simulink model "Model_TranslationEngine64"  (R2022b)
settings: Solver=FixedStepDiscrete  StartTime=0.0  StopTime=5  RelTol=1e-3  EnableMultiTasking=on
InitFcn:
  | % Initialize model
  | ModelSettings=BTConfig.GetModelSettings();
  | 
  | ModelSettings.Validate();
  | 
  | ModelInit;
  | 
  | 
  | % load library data
  | GainLibrary_data;
  | % Load saved values from partition process
  | CapturedConstMask.LoadMapFromFile(bdroot)
StartFcn:
  | % make sure all the simulated RTC requests are found
  | %RTC_SIM_OBJ.ValidateREQs();
undefined symbols (not defined in the file or in its folder): AA, BPLP, Column, NumHFRefBPF, NumHFRefLPF, NumMusicChannels, Row, VolumeMuteConfig
libraries: TuneVar x925, TOP x490, FeaturePath x111, CapturedConstLib x52
(part 1 of 34)
settings Model: Creator=kl13806  LastModifiedBy=mp55777
settings DataIOCC: ReturnWorkspaceOutputs=off
settings OptimizationCC: DefaultParameterBehavior=Inlined  DefaultUnderspecifiedDataType=single  EfficientTunableParamExpr=on
settings DebuggingCC: MergeDetectMultiDrivingBlocksExec=none  InheritedTsInSrcMsg=none  MultiTaskDSMMsg=none  ParameterPrecisionLossMsg=none  ParameterTunabilityLossMsg=error  UnconnectedInputMsg=warning  UnconnectedOutputMsg=warning  UnconnectedLineMsg=warning  UnknownTsInhSupMsg=none  SFUnexpectedBacktrackingDiag=warning  SFNoUnconditionalDefaultTransitionDiag=warning  SFExecutionAtInitializationDiag=none  SFMachineParentedDataDiag=warning
settings HardwareCC: ProdBitPerPointer=32  ProdBitPerSizeT=32  ProdBitPerPtrDiffT=32  ProdWordSize=32  ProdHWDeviceType=Intel->x86-32 (Windows32)  TargetBitPerPointer=64  TargetBitPerSizeT=64  TargetBitPerPtrDiffT=64  TargetLongLongMode=on  TargetIntDivRoundTo=Zero  TargetEndianess=LittleEndian  TargetWordSize=64  TargetHWDeviceType=MATLAB Host  ProdEqTarget=off
settings ModelReferenceCC: EnableRefExpFcnMdlSchedulingChecks=on  ModelReferenceNumInstancesAllowed=Single
settings SFSimCC: MATLABDynamicMemAlloc=off
settings RTWCC: Description=Embedded Coder (host-based shared library target)  SystemTargetFile=ert_shrlib.tlc  TLCOptions="-aTALARIA_ENGINE=\"Translation\""  TemplateMakefile=ert_default_tmf  RTWVerbose=off  RetainRTWFile=on  Toolchain=MinGW64 | gmake (64-bit Windows)  IncludeHyperlinkInReport=on
settings RTWCC: CustomHeaderCode=|
  | // Auto-generated code for model Model
  | /**** TOP TOKEN COMPATIBILITY HASH VALUES ****/
  | #define TOP_COMPAT {0x21D75357UL, 0x72F610E9UL, 0x8E520967UL, 0x8735CAA1UL, 0x168A3EA6UL}
  | #define TOP_COMPAT_NAME {"InputSelect", "PreAmp", "Near", "PostProcess", "TestRouter"}
  | #define TOP_COMPAT_NAME_HASH {0xF8044409UL, 0xC3A89EEBUL, 0xD67EB32FUL, 0x062DAD3BUL, 0x8CC5BE54UL}
  | /**** COMPAT HASH VALUES BY MODULE ****/
  | #define INPUTSELECT_TOP_COMPAT 0x21D75357UL
  | #define PREAMP_TOP_COMPAT 0x72F610E9UL
  | #define NEAR_TOP_COMPAT 0x8E520967UL
  | #define POSTPROCESS_TOP_COMPAT 0x8735CAA1UL
  | #define TESTROUTER_TOP_COMPAT 0x168A3EA6UL
  | /**** NAME HASH VALUES BY MODULE ****/
  | #define INPUTSELECT_TOP_NAME_HASH 0xF8044409UL
  | #define PREAMP_TOP_NAME_HASH 0xC3A89EEBUL
  | #define NEAR_TOP_NAME_HASH 0xD67EB32FUL
  | #define POSTPROCESS_TOP_NAME_HASH 0x062DAD3BUL
  | #define TESTROUTER_TOP_NAME_HASH 0x8CC5BE54UL
settings CodeAppCC: ForceParamTrailComments=on  IgnoreCustomStorageClasses=off  MaxIdLength=128  OperatorAnnotations=on  SimulinkDataObjDesc=on  SFDataObjDesc=on  MATLABFcnDesc=on  InsertBlockDesc=on  StateflowObjectComments=on  MATLABSourceComments=on
settings STFCustomTargetCC: TargetLangStandard=C99 (ISO)  MultiwordLength=256  ParMdlRefBuildCompliant=on  CompOptLevelCompliant=on  CombineOutputUpdateFcns=on  ERTCustomFileBanners=on  SupportContinuousTime=off  SupportNonInlinedSFcns=off  RemoveResetFunc=on  SupportVariableSizeSignals=on  MATLABClassNameForMDSCustomization=Simulink.SoftwareTarget.ERTCustomization  ModelStepFunctionPrototypeControlCompliant=on  UseToolchainInfoCompliant=on  SystemTargetFile=ert_shrlib.tlc
settings ERTTargetCC: TargetLangStandard=C99 (ISO)  ConcurrentExecutionCompliant=off  SupportVariableSizeSignals=on  CPPClassGenCompliant=off  InlinedParameterPlacement=NonHierarchical  ERTCustomFileTemplate=translation_dll.tlc  IndentStyle=Allman  IndentSize=4

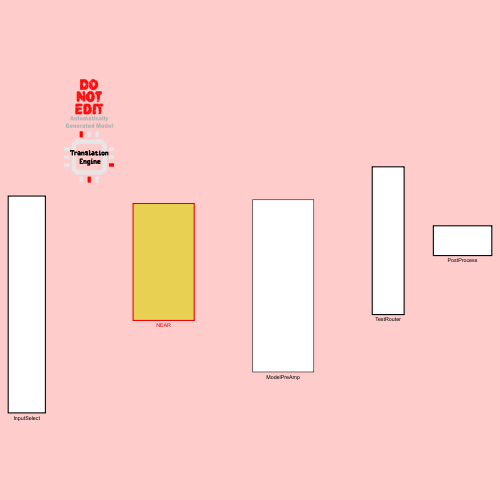
[thumbnail: Simulink's stored preview of the top-level diagram]
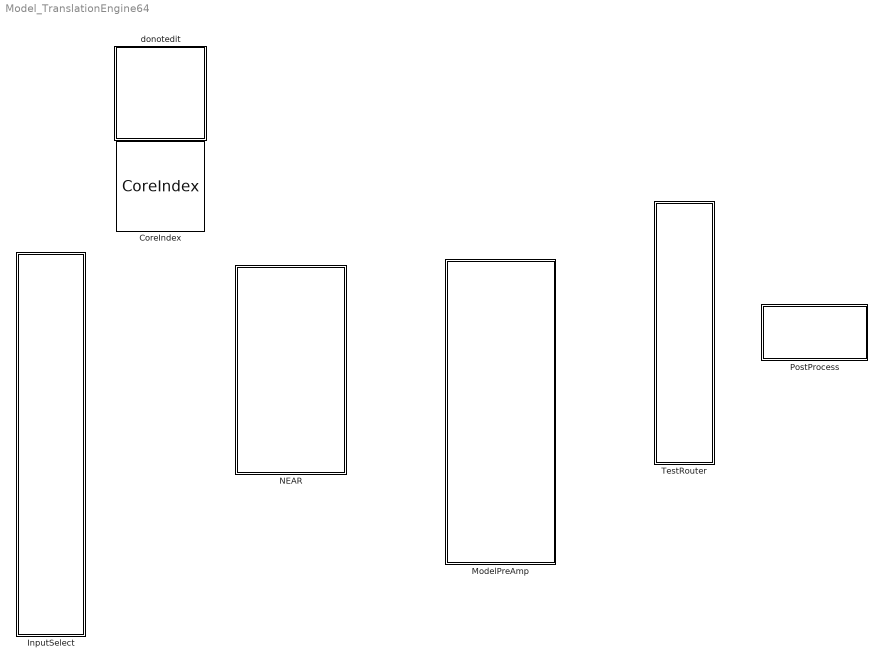
== system Model_TranslationEngine64 ==
  CoreIndex : FeaturePath/CoreIndex  Role=Translation Engine  CoreIndex=9  Config=[]  AddressingMode=Indirect core determination via table lookup (i.e. use Partition blocks)  CrossCoreApi=None  CrossCoreAllocation=None  CrossCoreSampleTime=-1  BasePeriod=[]  TriggerInit=[440 234 535 331]
      settings: SourceProductName=Bose Talaria
  InputSelect : Subsystem  TreatAsAtomicUnit=on  mask{Config=ModelSettings.InputSelect}
      mask prompts: Config "InputSelectConfig"
      settings: RTWSystemCode=Nonreusable function
  ModelPreAmp : Subsystem  mask{Config=ModelSettings.ModelPreAmp}
      mask prompts: Config "PreAmpConfig"
  NEAR : Subsystem  TreatAsAtomicUnit=on  mask{Config=ModelSettings.NearConfig}
      mask prompts: Config "NearConfig"
  PostProcess : Subsystem  TreatAsAtomicUnit=on  mask{Config=ModelSettings.PostProcess}
      mask prompts: Config "PostProcessConfig"
  TestRouter : Subsystem  TreatAsAtomicUnit=on  mask{Config=ModelSettings.TestRouter}
      mask prompts: Config "TestRouterConfig"
  donotedit : Subsystem
      settings: OpenFcn=Model
      mask Display: image('DoNotEdit.svg');

== system Model_TranslationEngine64/InputSelect ==
  FeaturePath : FeaturePath/FeaturePath  FeatureName=InputSelect  IsGroup=on  GroupNumber=0  IsModule=on  TriggerInit=[105 216 220 329]
      settings: SourceProductName=Bose Talaria
  Router : Subsystem  mask(Blocklib Router){Config=Config.RouterCfg, FeatureName=RouterCfg}
      mask prompts: Config "RouterConfig"; FeatureName "Feature path name:"
      mask help: This block allows the user to route X input channels to Y output channels. Enter a value of 0 to "zero out" the specific channel
      mask init:
      | blkh=gcbh;
      | Config=BTConfig.Assert(blkh,Config);
      | 
      | Config.Validate();
      | BTConfig.InitSetFeatureIfPresent(blkh,'FeatureName');
      mask Callback Config: BTConfig.CallbackHideIfPresent(gcbh,{'FeatureName'});
      mask TypeOptions FeatureName: FeaturePath/FeatureName
      mask Display: image('routerIcon.png');

== system Model_TranslationEngine64/ModelPreAmp ==
  DecRate : Subsystem
  FeaturePath : FeaturePath/FeaturePath  FeatureName=PreAmp  IsGroup=on  GroupNumber=2  IsModule=on  TriggerInit=[-135 -246 -20 -139]
      settings: SourceProductName=Bose Talaria
  PreAmpPart1 : Subsystem  TreatAsAtomicUnit=on
      settings: RTWSystemCode=Nonreusable function  FunctionWithSeparateData=on

== system Model_TranslationEngine64/NEAR ==
  FeaturePath : FeaturePath/FeaturePath  FeatureName=Near  IsGroup=on  GroupNumber=1  IsModule=on  TriggerInit=[15 -306 130 -199]
      settings: SourceProductName=Bose Talaria
  Near1p1 : Subsystem  mask{Config=Config.Near}
      mask prompts: Config "Near1p1Config"
      mask init:
      | blkh=gcbh;
      | Config=BTConfig.Assert(blkh,Config);
      | % sample_rate_in_hertz                        = near.sample_rate_in_hertz;
      | % frame_size                                  = near.frame_size;
      | % ann_sysin_channel_count                     = near.ann_sysin_channel_count;
      | % front_peripheral_channel_count              = near.front_peripheral_channel_count;
      | % NEAR1p1FrontPeripheralChannelCountFullRate  = near.NEAR1p1FrontPeripheralChannelCountFullRate;
      | % NearWbAnnCount                              = near.NearWbAnnCount;
      | % headrest_count                              = near.headrest_count;
      | % channels_per_headrest                       = near.channels_per_headrest;
      | % decimation_factor                           = near.decimation_factor;
      | % rear_channel_count                          = near.rear_channel_count;
      | % vm                                          = near.vm;
      | % decimated_frame_size                        = near.decimated_frame_size;
      | % decimated_sample_rate_in_hertz              = near.decimated_sample_rate_in_hertz;
      | Config.Validate();
      | Config.DoMaskInit(blkh);

== system Model_TranslationEngine64/PostProcess ==
  FeaturePath : FeaturePath/FeaturePath  FeatureName=PostProcess  IsGroup=on  GroupNumber=3  IsModule=on  TriggerInit=[85 -186 200 -79]
      settings: SourceProductName=Bose Talaria
  PostProcess : Subsystem  TreatAsAtomicUnit=on
      settings: RTWSystemCode=Nonreusable function  RTWFcnNameOpts=Use subsystem name  RTWFileNameOpts=Use subsystem name  FunctionWithSeparateData=on

== system Model_TranslationEngine64/TestRouter ==
  ASDRouter : Subsystem  mask{frameSize=Config.FrameSize, nChanOut=Config.NumChanOut, mainSelect=Config.MainSelect, numMainCh=Config.NumMainCh, mainGain=Config.MainGain, enableAux=Config.EnableAux, numAux=Config.NumAux, auxGain=Config.AuxGain}
      mask prompts: frameSize "Frame Size (L)"; nChanOut "Number of Output Channels"; mainSelect "Main Channel Select Vector"; numMainCh "Number of Main Channels"; mainGain "Main gain for each output channel"; enableAux "Enable Aux input sources"; numAux "Number of Aux Channels"; auxGain "Aux gain for each output channel for each Aux source"
      mask init:
      | blkh = gcbh;
      | % Copy discrete mask parameters into a classdef object
      | InnerLinkConfig = AsdRouterConfig;
      | InnerLinkConfig.FrameSize = frameSize;
      | InnerLinkConfig.NumChanOut = nChanOut;
      | InnerLinkConfig.MainSelect = mainSelect;
      | InnerLinkConfig.NumMainCh = numMainCh;
      | InnerLinkConfig.MainGain = mainGain;
      | InnerLinkConfig.EnableAux = enableAux;
      | InnerLinkConfig.NumAux = numAux;
      | InnerLinkConfig.AuxGain = auxGain;
  FeaturePath : FeaturePath/FeaturePath  FeatureName=TestRouter  IsGroup=on  GroupNumber=5  IsModule=off  TriggerInit=[290 -166 405 -59]
      settings: SourceProductName=Bose Talaria
  TuneTOP : Subsystem  mask(Talaria Trivial Tune TOP){TriggerInit=[175 117 345 173], TopName=AuxSelect, TuneName=AuxSelect, DataTypeOut=int32, MaskValue=Config.MainGain, TunabilityNumber=1, MinValue=[], MaxValue=[], BankNumber=0, PreOverlay=false, PostOverlay=false, UseSameName=on}
      mask prompts: TriggerInit "Hidden: MoveFcn redraw"; TopName "Name:"; TuneName "Name of TuneVar:"; DataTypeOut "Data type:"; MaskValue "Default Value:"; TunabilityNumber "Tunability:"; MinValue "Min Value:"; MaxValue "Max Value:"; BankNumber "Target memory bank number:"; PreOverlay "Requires pre-overlay action:"; PostOverlay "Requires post-overlay action:"; UseSameName "Use same name for tune variable and TOP"
      mask help: The TuneTOP block encapsultes a Target Overlay Parameter, a Tune Variable, and a Trivial Translation between them.
      mask init:
      | [ok,activeTopPath,activeTunePath] = TuneTOP_Mask.Init(gcbh);
      settings: MoveFcn=TuneTOP_Mask.CB_TriggerInit(gcbh);
      mask Callback TriggerInit: TuneTOP_Mask.CB_TriggerInit(gcbh);
      mask TypeOptions TopName: TOP/TopName
      mask TypeOptions TuneName: Tune Variable/TuneName
      mask TypeOptions DataTypeOut: TOP/DataTypeOut
      mask TypeOptions MaskValue: Tune Variable/MaskValue
      mask TypeOptions TunabilityNumber: Tune Variable/TunabilityNumber
      mask Callback TunabilityNumber: TuneVarMask.CB_TunabilityNumber(gcbh);
      mask TypeOptions MinValue: Tune Variable/MinValue
      mask TypeOptions MaxValue: Tune Variable/MaxValue
      mask TypeOptions BankNumber: TOP/BankNumber
      mask TypeOptions PreOverlay: TOP/PreOverlay
      mask TypeOptions PostOverlay: TOP/PostOverlay
      mask Callback UseSameName: TuneTOP_Mask.CB_UseSameName(gcbh);
      mask DialogControl toolPanel Prompt: Tuning Tool Hints
      mask DialogControl DescriptionGroup Prompt: Description
      mask DialogControl EditDescription Prompt: Edit Description
      mask DialogControl EditDescription Callback: TuneTOP_Mask.CB_EditDescription(gcbh);
      mask DialogControl TunabilityText Prompt: Easy: Changes nearly every tuning.
      mask DialogControl AdvancedPanel Prompt: Advanced
      mask DialogControl ConvertToFullTranslation Prompt: Irreversible conversion to full translation
      mask DialogControl ConvertToFullTranslation Callback: TuneTOP_Mask.CB_ConvertToFullTranslation(gcbh);
      mask DialogControl ErrorContainer Prompt: Error Messages
      mask DialogControl ErrorText Prompt: Default value cannot be empty. Tune variables must have non-zero dimensions.
      mask Display:
      | % retrieve icon definition
      | [path,w,h] = TuneTOP_Mask.Icon();
      | 
      | % retrieve the block's pixel size
      | pos = get(gcbh,'position');
      | bw = pos(3) - pos(1);
      | bh = pos(4) - pos(2);
      | 
      | % draw centered icon
      | xAdj = bw/2 - w/2 + 5;
      | yAdj = bh/2 - h/2 + 4;
      | for i=1:length(path)
      | 	patch(path(i).x+xAdj, path(i).y+yAdj, path(i).rgb);
      | end
      | 
      | % show the top name or an X
      | if (exist('ok','var') && ok)
      | 	text(bw*0.5, bh*0.2, activeTopPath, 'horizontalAlignment', 'center');
      | 	patch(0,0,[1 1 1]);
      | 	patch(bw,bh,[1 1 1]);
      | else
      | 	tx=bw*0.03;
      | 	ty=bh*0.03;
      | 	patch([0 tx bw bw-tx], [ty 0 bh-ty bh], [1 0 0]);
      | 	patch([0 bw-tx bw tx], [bh-ty 0 ty bh], [1 0 0]);
      | end

== system Model_TranslationEngine64/donotedit ==

== system Model_TranslationEngine64/InputSelect/Router ==
  FeaturePath : FeaturePath/FeaturePath  FeatureName=RouterCfg  IsGroup=off  GroupNumber=-1  IsModule=off  TriggerInit=[615 164 730 271]
      settings: SourceProductName=Bose Talaria
  TOP : TOP/TOP  TriggerInit=[660 425 805 485]  TopName=OutMap  DataTypeOut=int32  BankNumber=0  PreOverlay=false  PostOverlay=false  Role=Automatic
      settings: SourceProductName=Bose Talaria
  TranslateTrigger : TuneVar/TranslateTrigger  TriggerInit=[526 305 564 360]
      settings: SourceProductName=Bose Talaria
  Trivial Translation : MATLAB Function  TreatAsAtomicUnit=on  mask{nInRouterMask=Config.NumIn}
      mask prompts: nInRouterMask "Num Input"
  TuneVarRouterMap : TuneVar/TuneVar  TuneName=Map  SpecifyMaxSize=on  VariableDim=2 (Column)  MaxSize=[1 Config.NumOut]  TunabilityNumber=1  MinValue=[]  MaxValue=[]  TriggerInit=[250 430 420 480]  MaskValue=Config.DefaultOutputMap
      settings: SourceProductName=Bose Talaria
  wires:
  TranslateTrigger/1 -> Trivial Translation/Trigger
  Trivial Translation/1(OutMap) -> TOP/1
  TuneVarRouterMap/1 -> Trivial Translation/1(Map)  "Map"

== system Model_TranslationEngine64/ModelPreAmp/DecRate ==
  AudioPilot35 : Subsystem  TreatAsAtomicUnit=on
      settings: RTWFcnNameOpts=Use subsystem name  RTWFileNameOpts=Use subsystem name  FunctionWithSeparateData=on
  Medusa5H1 : Subsystem

== system Model_TranslationEngine64/ModelPreAmp/PreAmpPart1 ==
  Bass : Subsystem  mask(Blocklib Tone){FeatureName=Bass, Config=Config.Bass, TriggerInit=[215 80 320 140]}
      mask prompts: FeatureName "Feature path name:"; Config "ToneConfig"; TriggerInit "Hidden: MoveFcn redraw"
      mask help: The tone block performs the treble and bass tone controls across multiple channels via a 1st order filter.
      mask init:
      | blkh=gcbh;
      | Config=BTConfig.Assert(blkh,Config);
      | 
      | BTConfig.InitSetFeatureIfPresent(blkh,'FeatureName');
      | Config.Validate();
      | ToneMask.Init(blkh);
      mask Help:
      | The tone block performs the treble and bass tone controls across multiple channels via a 1st order filter. The treble/ bass content can either be 'boosted' or 'cut' depending on the value of the gain. Different filters can be used for the boost and cut regions, each with its own cut-off frequency.
      | 
      | MASK PARAMETERS:
      | - Different filter coefficients can be applied for the boost and cut regions
      | - The maximum boost/ cut can be specified (typically 20 dB and -20 dB)
      | - The offset and scale values determine the piecewise linear curve that maps the index to the gain (typically 128 and 127 respectively)
      | 
      | RTC CONTROL:
      | Run time control is available to dynamically change the gain to be applied to the treble/bass content. An index (typically between 0-255) can be provided along with a ramp time and rate (rate gets precedence).
      | RTC_SIM_OBJ.AddREQ( 'TrebleBassSet', 0.6, [0005,  <tone_index>, <ramp_db_per_second>, <ramp_time>]);
      | E.g., RTC_SIM_OBJ.AddREQ( 'TrebleBassSet', 0.6, [0005,  50, 0, 50]);
      mask TypeOptions FeatureName: FeaturePath/FeatureName
      mask Callback Config: BTConfig.CallbackHideIfPresent(gcbh,{'FeatureName'});
      mask Callback TriggerInit: ToneMask.CB_TriggerInit(gcbh);
      mask Display:
      | [path w h] = IconToneMask();
      | 
      | % retrieve the block's pixel size
      | pos = get(gcbh,'position');
      | bw = pos(3) - pos(1);
      | bh = pos(4) - pos(2);
      | 
      | % draw centered icon
      | xAdj = bw/2 - w/2;
      | yAdj = bh/2 - h/2 + 4;
      | for i=1:length(path)
      | 	patch(path(i).x+xAdj, path(i).y+yAdj, path(i).rgb);
      | end
      | 
      | % place feature name text
      | 	text(bw*0.5, 0, [FeatureName '\n\n'], 'horizontalAlignment', 'center');
  Midrange : Subsystem  mask(Blocklib Midrange){FeatureName=Midrange, Config=Config.Midrange}
      mask prompts: FeatureName "Feature path name:"; Config "MidrangeConfig"
      mask help: The midrange block performs tone controls across midrange frequencies across multiple channels via a 2nd order IIR filter.
      mask init:
      | blkh=gcbh;
      | Config=BTConfig.Assert(blkh,Config);
      | MaskBlockHandle = gcbh;
      | 
      | MidrangeMask.Init(blkh);
      | 
      | % Set boundary conditions
      | rampRateBounds = [5,50000];
      | rampTimeBounds = [1,3000];
      | 
      | BTConfig.InitSetFeatureIfPresent(blkh,'FeatureName');
      | Config.Validate();
      mask Help:
      | The midrange block performs tone controls across midrange frequencies across multiple channels via a 2nd order IIR filter. The midrange content can either be 'boosted' or 'cut' depending on the value of the gain. Different filters can be used for the boost and cut regions, each with its own center frequency and Q value.
      | 
      | MASK PARAMETERS:
      | - Different filter coefficients can be applied for the boost and cut regions (typical center frequency - 775 Hz, Q - 0.9)
      | - The maximum boost/ cut can be specified (typically 20 dB and -20 dB)
      | - The offset and scale values determine the piecewise linear curve that is used to compute the gain (typically 128 and 127 respectively)
      | 
      | RTC CONTROL:
      | Run time control is available to dynamically change the gain to be applied to the midrange content. An index (typically between 0-255) can be provided along with a ramp time and rate (rate gets precedence).
      | RTC_SIM_OBJ.AddREQ( 'MidrangeSet', 0.6, [0005,  <midrange_index>, <ramp_db_per_second>, <ramp_time>]);
      | E.g., RTC_SIM_OBJ.AddREQ( 'MidrangeSet', 0.6, [0005,  50, 0, 50]);
      mask TypeOptions FeatureName: FeaturePath/FeatureName
      mask Callback Config: BTConfig.CallbackHideIfPresent(gcbh,{'FeatureName'});
      mask Display:
      | [path w h] = IconToneMask();
      | 
      | % retrieve the block's pixel size
      | pos = get(gcbh,'position');
      | bw = pos(3) - pos(1);
      | bh = pos(4) - pos(2);
      | 
      | % draw centered icon
      | xAdj = bw/2 - w/2;
      | yAdj = bh/2 - h/2 + 4;
      | for i=1:length(path)
      | 	patch(path(i).x+xAdj, path(i).y+yAdj, path(i).rgb);
      | end
      | 
      | % place feature name text
      | 	text(bw*0.5, 0, ['\n' FeatureName '\n\n'], 'horizontalAlignment', 'center');
  NEARPreAmp : Subsystem  mask(PreAmp){Config=Config.NearPreAmpConfig}
      mask prompts: Config "PreAmpConfig"
      mask help:
      | This mask allows the setting of parameters for the PreAmp model. Model parameters are set by association with a class instance of PreAmpClass.m.
      |
      | See 'Help' for details.
      mask init:
      | blkh=gcbh;
      | Config=BTConfig.Assert(blkh,Config);
      | 
      | Config.Validate();
      | Config.DoMaskInit(blkh);
      mask Help:
      | Model parameters are set by a class instance in the base workspace.
      | 
      | To configure the model:
      | 1 - Create an instance of PreAmpClass.m in the base workspace.
      | 2 - Set the 'Class Instance' mask parameter to the instance created in step 1.
  Treble : Subsystem  mask(Blocklib Tone){FeatureName=Treble, Config=Config.Treble, TriggerInit=[395 80 500 140]}
      mask prompts: FeatureName "Feature path name:"; Config "ToneConfig"; TriggerInit "Hidden: MoveFcn redraw"
      mask help: The tone block performs the treble and bass tone controls across multiple channels via a 1st order filter.
      mask init:
      | blkh=gcbh;
      | Config=BTConfig.Assert(blkh,Config);
      | 
      | BTConfig.InitSetFeatureIfPresent(blkh,'FeatureName');
      | Config.Validate();
      | ToneMask.Init(blkh);
      mask Help:
      | The tone block performs the treble and bass tone controls across multiple channels via a 1st order filter. The treble/ bass content can either be 'boosted' or 'cut' depending on the value of the gain. Different filters can be used for the boost and cut regions, each with its own cut-off frequency.
      | 
      | MASK PARAMETERS:
      | - Different filter coefficients can be applied for the boost and cut regions
      | - The maximum boost/ cut can be specified (typically 20 dB and -20 dB)
      | - The offset and scale values determine the piecewise linear curve that maps the index to the gain (typically 128 and 127 respectively)
      | 
      | RTC CONTROL:
      | Run time control is available to dynamically change the gain to be applied to the treble/bass content. An index (typically between 0-255) can be provided along with a ramp time and rate (rate gets precedence).
      | RTC_SIM_OBJ.AddREQ( 'TrebleBassSet', 0.6, [0005,  <tone_index>, <ramp_db_per_second>, <ramp_time>]);
      | E.g., RTC_SIM_OBJ.AddREQ( 'TrebleBassSet', 0.6, [0005,  50, 0, 50]);
      mask TypeOptions FeatureName: FeaturePath/FeatureName
      mask Callback Config: BTConfig.CallbackHideIfPresent(gcbh,{'FeatureName'});
      mask Callback TriggerInit: ToneMask.CB_TriggerInit(gcbh);
      mask Display:
      | [path w h] = IconToneMask();
      | 
      | % retrieve the block's pixel size
      | pos = get(gcbh,'position');
      | bw = pos(3) - pos(1);
      | bh = pos(4) - pos(2);
      | 
      | % draw centered icon
      | xAdj = bw/2 - w/2;
      | yAdj = bh/2 - h/2 + 4;
      | for i=1:length(path)
      | 	patch(path(i).x+xAdj, path(i).y+yAdj, path(i).rgb);
      | end
      | 
      | % place feature name text
      | 	text(bw*0.5, 0, [FeatureName '\n\n'], 'horizontalAlignment', 'center');

== system Model_TranslationEngine64/NEAR/Near1p1 ==
  DrProc : Subsystem
  FrProc : Subsystem
  LocRamper : Subsystem
  NearBandSplit : Subsystem  mask(NEAR BandSplit){Config=Config.NearBandSplit}
      mask prompts: Config "NearBandSplitConfig"
      mask help:
      | This mask allows the setting of parameters for version 1.1 of the NEAR BandSplit model.
      | Model parameters are set by a class instance in the base workspace.
      |
      | See 'Help' for details.
      mask init:
      | blkh=gcbh;
      | Config=BTConfig.Assert(blkh,Config);
      | 
      | Config.Validate();
      | Config.DoMaskInit(blkh);
      mask Help:
      | Defining model parameters:
      | The model parameters are set by the conents of an instance of BandSplitConfig.m.
      | 
      | To set model parameters:
      | 1-Create an instance of BandSplitConfig.m in the base workspace.
      | 2-In the model mask, set the 'Class instance' parameter to the name of the class instance in the base workspace.
  VolumeMute : Subsystem  mask{Config=Config.VolumeMute}
      mask prompts: Config "VolumeMuteConfig"
      mask init:
      | blkh=gcbh;
      | Config=BTConfig.Assert(blkh,Config);
      | 
      | Config.Validate();
      | Config.DoMaskInit(blkh);

== system Model_TranslationEngine64/PostProcess/PostProcess ==
  Limiter : Subsystem
  Mute : Subsystem
  PostLimiterEQ : Subsystem
  Soft Clipper : Subsystem

== system Model_TranslationEngine64/TestRouter/ASDRouter ==
  InnerLink : Subsystem  mask(Blocklib AsdRouter){Config=InnerLinkConfig, FeatureName=ASDRouter}
      mask prompts: Config "AsdRouterConfig"; FeatureName "Feature path name:"
      mask init:
      | blkh=gcbh;
      | Config=BTConfig.Assert(blkh,Config);
      | Config.Validate();
      | BTConfig.InitSetFeatureIfPresent(blkh,'FeatureName');
      | 
      | % Most significant bit (MSB) of RTC parameters is used to switch between RTC
      | % & TuneTOP configurations. If MSB of any RTC parameter is set to '1' means
      | % TuneTOP values will be used. By default TuneTOP configurations are to be used, so MSB of all RTC parameters
      | % is set to '1' by initializing with negative number.
      | mainSelectRTCInit = -ones(1,Config.NumChanOut);
      | enableAuxRTCInit = -ones(1,length(Config.NumAux));
      | auxSelectRTCInit = -ones(1,Config.NumChanOut*length(Config.NumAux));
      mask Callback Config: BTConfig.CallbackHideIfPresent(gcbh,{'FeatureName'});
      mask TypeOptions FeatureName: FeaturePath/FeatureName

== system Model_TranslationEngine64/TestRouter/TuneTOP ==
  TOP : TOP/TOP  TriggerInit=[440 20 585 80]  TopName=AuxSelect  DataTypeOut=int32  BankNumber=BankNumber  PreOverlay=PreOverlay  PostOverlay=PostOverlay  Role=Automatic
      settings: SourceProductName=Bose Talaria
  TrivialTranslation : TuneVar/TrivialTranslation  TriggerInit=[300 28 350 72]
      settings: SourceProductName=Bose Talaria
  Tune Variable : TuneVar/TuneVar  TuneName=AuxSelect  SpecifyMaxSize=off  VariableDim=1 (Row)  MaxSize=[1 1]  TunabilityNumber=1  MinValue=MinValue  MaxValue=MaxValue  TriggerInit=[20 25 190 75]  MaskValue=MaskValue
      settings: SourceProductName=Bose Talaria
  wires:
  Tune Variable/1 -> TrivialTranslation/1  "AuxSelect"
  TrivialTranslation/1 -> TOP/1

== system Model_TranslationEngine64/ModelPreAmp/DecRate/AudioPilot35 ==
  Audiopilot_3_5 : Subsystem  mask(AudioPilot 3.5){FeatureName=Audiopilot, InputAudioMode=Stereo - 2 Channels, NoiseEstimationMode=Regular, IncludeSpumTails=off, IncludeIgnoreMicFlag=off, Config=Config.Audiopilot}
      mask prompts: FeatureName "Feature Name:"; InputAudioMode "Input Audio Mode"; NoiseEstimationMode "Mode"; IncludeSpumTails "Include SPUM Tails as Reference Channels for High-Frequency Noise Estimator"; IncludeIgnoreMicFlag "Include Ignore Microphone Flag as Input"; Config "Audiopilot_3_5Config"
      mask help:
      | This is the top level model implementing AudioPilot 3.5.
      | It is configurable to accommodate both stereo inputs and surround inputs.  It can also reconfigure itself to become a speed-only implementation. For the regular implementation, there are two options. One is to allow a flag signal to instruct the algorithm to ignore the microphone signal; the other is to include in the set of "high-passed" reference channels the 2 channels representing the SPUM tails from the Medusa Upmixer.
      | Build Time Configuration settings typically set for this block include the frame size and the sample rate of the input audio. Other options include the type of code generation and whether all RTC blocks will generate a response.
      mask init:
      | blkh = gcbh;
      | 
      | Config = BTConfig.Assert(blkh,Config);
      | Config.Validate();
      | 
      | FrameSize = Config.FrameSize;
      | SampleRate = Config.SampleRateHz;
      |  
      | % Make the choice for the Noise Estimation Variant
      | Audiopilot_3_5Mask.ConfigureVariant(blkh,NoiseEstimationMode);
      | 
      | % Set up the number of audio channels for each input
      | [NumMicChannels,NumMusicChannels, ...
      |     NumHFRefLPF,NumHFRefBPF,NumLFRef] = ...
      |     Audiopilot_3_5Mask.ChannelSetUp(blkh,InputAudioMode,...
      |                 NoiseEstimationMode,IncludeSpumTails);
      | 
      | % Configure RTC responses            
      | Audiopilot_3_5Mask.ConfigureRtcResponses(blkh,...
      |                 Config.EnableRtcResponse)           
      | 
      | % Configure the Model according to Mask Parameters   
      | Audiopilot_3_5Mask.ConfigureModel(blkh,InputAudioMode,...
      |     NoiseEstimationMode,IncludeIgnoreMicFlag);
      | 
      | BTConfig.InitSetFeatureIfPresent(blkh,'FeatureName');
      mask TypeOptions FeatureName: FeaturePath/FeatureName
      mask TypeOptions InputAudioMode: Stereo - 2 Channels | Surround - 6 Channels
      mask TypeOptions NoiseEstimationMode: Regular | Speed Only
      mask Callback NoiseEstimationMode: Audiopilot_3_5Mask.NoiseEstimationModeCallBack(gcbh);
      mask Callback Config: BTConfig.CallbackHideIfPresent(gcbh,{'FeatureName'});
      mask DialogControl DTCTitle Prompt: <b> Design Time Configuration </b>
      mask DialogControl NoiseEstimationBox Prompt: Noise Estimation
      mask DialogControl BTCTitle Prompt: <b> Build Time Configuration </b>
  EntertainmentLevelDetection : Subsystem  mask(Level Detector for AudioPilot, Dyanmic EQ, Fan and Boost-on-Demand){NumInputChannels=Config.AudiopilotNumMusicIn, FANEnable=off, BODEnable=off, Config=Config.LDCfg}
      mask prompts: NumInputChannels "Number of Input Channels"; FANEnable "FAN (amplifier fan control)"; BODEnable "BOD (boost on demand)"; Config "EntertainmentLevelDetectionConfig"
      mask help: This block performs level detection, separately and independently, for various features. The features, AudioPilot and Dynamic Equalization, are always included. The other features, Amplifier Fan Control, and Boost on Demand, are optional. The block is designed to accept as input the entertainment audio channels before volume control was applied. The volume setting, in linear, forms a different input.
      mask init:
      | blkh = gcbh;
      | 
      | Config = BTConfig.Assert(blkh,Config);
      | Config.Validate();
      | 
      | SampleRate = Config.SampleRateHz;
      | FrameSize = Config.FrameSize;
      | FrameRate = Config.FrameRateHz;
      | MaxMusicDelay = Config.MaxMusicDelay;
      | MaxMusicDelayPerChannel = floor(MaxMusicDelay/NumInputChannels);
      | 
      | EntertainmentLevelDetectionMask.ConfigureAdditionalLevelDetectors ...
      |     (blkh,FANEnable,BODEnable)
      mask Help:
      | This block performs level detection for various features.
      | 
      | Arguments for this block:
      | 
      | Configuration
      | The block can be configured using a object of class, EntertainmentLevelDetectionConfig.  If the "use Default Configuration Only" box is checked, then this option is disabled.
      | 
      | Additional Level Estimates
      | FAN (amplifier fan control)
      | BOD (boost on demand)
      | 
      | System Definitions
      | Sample Rate --- Fs
      | Frame Size --- frameSize
      | Maximum Delay for the Music --- maxMusicDelay
      mask DialogControl DTC Prompt: Design Time Configuration
      mask DialogControl AdditionalGroup Prompt: Additional Level Estimates
      mask DialogControl BTC Prompt: Build Time Configuration
  Volume : Subsystem  mask(Blocklib Volume){FeatureName=VolumeCfg, Config=Config.VolumeCfg, EnableGainOut=on, TriggerInit=[100 -29 180 24]}
      mask prompts: FeatureName "Feature path name:"; Config "VolumeConfig"; EnableGainOut "Enable gain output"; TriggerInit "Hidden: MoveFcn redraw"
      mask help: This volume signal block includes receipt of volume level (via RTC) as well as tuning variables to calibrate a gain table that maps 8-bit integer volume index (from RTC) to float decibels.
      mask init:
      | blkh=gcbh;
      | Config=BTConfig.Assert(blkh,Config);
      | 
      | % Set boundary conditions
      | rampRateBounds = [5,50000];
      | rampTimeBounds = [1,3000];
      | BTConfig.InitSetFeatureIfPresent(blkh,'FeatureName');
      | Config.Validate();
      | 
      | EnableBlockPort(blkh,'gain out',EnableGainOut);
      settings: MoveFcn=VolumeMask.CB_TriggerInit(gcbh);
      mask Help:
      | This block allows a ramped change in volume using rgainy block.
      | - The initial gain to be applied to the input audio can be set (typically 0)
      | 
      | RTC CONTROL:
      | Run time control is available to dynamically mute the audio. The volume index can be provided (typically between 0-255), along with a ramp time and rate (rate gets precedence).
      | RTC_SIM_OBJ.AddREQ( 'VolumeSet', 0.6, [0005,  <volume_index>, <ramp_db_per_second>, <ramp_time>]);
      | E.g., RTC_SIM_OBJ.AddREQ( 'VolumeSet', 0.7, [0005, 255, 0, 50]);
      mask TypeOptions FeatureName: FeaturePath/FeatureName
      mask Callback Config: BTConfig.CallbackHideIfPresent(gcbh,{'FeatureName'});
      mask Callback TriggerInit: VolumeMask.CB_TriggerInit(gcbh);
      mask Display:
      | [path,w,h] = IconVolumeMask();
      | 
      | % work in pixels since the icon does not scale
      | pos = get(gcbh,'position');
      | bw = pos(3) - pos(1);
      | bh = pos(4) - pos(2);
      | 
      | % Draw centered icon
      | xAdj = bw/2 - w/2;
      | yAdj = bh/2 - h/2;
      | for i=1:length(path)
      |     if (path(i).rgb(1) >= 0)
      |         patch(path(i).x+xAdj, path(i).y+yAdj, path(i).rgb);
      |     end
      |     if (path(i).stroke(1) >= 0)
      |         plot(path(i).x+xAdj, path(i).y+yAdj);
      |     end
      | end
      | 
      | % Display some text
      | text(bw/2, bh/2,FeatureName, ...
      |     'horizontalAlignment','center', ...
      |     'VerticalAlignment','middle');

== system Model_TranslationEngine64/ModelPreAmp/DecRate/Medusa5H1 ==
  Balance : Subsystem  TreatAsAtomicUnit=on
  MedusaHoligram : Subsystem  mask{config=Config.MedusaConfig, ConfigBTC=Config.MedusaBTC, vlsConfigStruct=Config.VLSConfig}
      mask prompts: config "Medusa config struct name:"; ConfigBTC "Medusa BTC config struct name:"; vlsConfigStruct "VLS config struct name:"
      mask init:
      | tailCompEQ = config.tailCompEQ;
      | HRDelayConfig = vlsConfigStruct.HeadrestDelayConfig;
  MedusaPostHoligram : Subsystem  TreatAsAtomicUnit=on
  NearWiggleFilters : Subsystem  TreatAsAtomicUnit=on
  SleepingBeauty : Subsystem  TreatAsAtomicUnit=on
  VLS : Subsystem  TreatAsAtomicUnit=on  mask(Virtual Loudspeaker){configStruct=Config.VLSConfig}
      mask prompts: configStruct "Config struct name:"
      mask init:
      | numGains = configStruct.VLSGainsConfig.numGains;
      settings: RTWSystemCode=Nonreusable function  RTWFcnNameOpts=Use subsystem name  RTWFileNameOpts=Use subsystem name  FunctionWithSeparateData=on
